simulink model "Simulink_System3"  (R2020a)
settings: Solver=VariableStepAuto  StartTime=0.0  StopTime=3  MaxStep=0.001  RelTol=1e-3
undefined symbols (not defined in the file): a, k3, kcA3, kcDO3, kcSO3, kdA3, kdDO3, kdSO3, kiA3, kiDO3, kiSO3
libraries: cstblocks x5, simulink x1
settings Model: Creator=beto1  LastModifiedBy=beto1

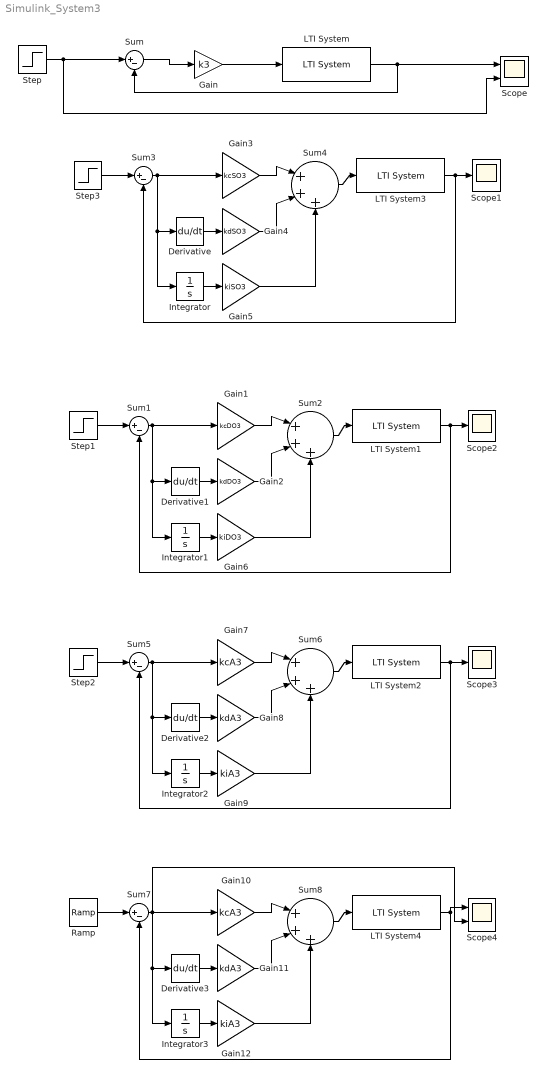
== system Simulink_System3 ==
  Derivative{,1..3} (4 alike) : Derivative
  Gain : Gain  Gain=k3
  Gain1 : Gain  Gain=kcDO3
  Gain10 : Gain  Gain=kcA3
  Gain11 : Gain  Gain=kdA3
  Gain12 : Gain  Gain=kiA3
  Gain2 : Gain  Gain=kdDO3
  Gain3 : Gain  Gain=kcSO3
  Gain4 : Gain  Gain=kdSO3
  Gain5 : Gain  Gain=kiSO3
  Gain6 : Gain  Gain=kiDO3
  Gain7 : Gain  Gain=kcA3
  Gain8 : Gain  Gain=kdA3
  Gain9 : Gain  Gain=kiA3
  Integrator{,1..3} (4 alike) : Integrator
  LTI System{,1..4} (5 alike) : cstblocks/LTI System  sys=G3  IC=[]
  Ramp : simulink/Sources/Ramp  slope=a  start=0  InitialOutput=0
  Scope : Scope  NumInputPorts=2
  Scope1 : Scope
  Scope2 : Scope
  Scope3 : Scope
  Scope4 : Scope  NumInputPorts=2
  Step : Step  Time=0  SampleTime=0
  Step1 : Step  Time=0  After=8  SampleTime=0
  Step2 : Step  Time=0  After=8  SampleTime=0
  Step3 : Step  Time=0  After=8  SampleTime=0
  Sum{,1,3,5,7} (5 alike) : Sum  Inputs=|+-
  Sum{2,4,6,8} (4 alike) : Sum  Inputs=|+++
  wires:
  Step/1 -> Sum/1, Scope/2
  LTI System/1 -> Sum/2, Scope/1
  Sum/1 -> Gain/1
  Gain/1 -> LTI System/1
  Gain4/1 -> Sum4/2
  Step3/1 -> Sum3/1
  Sum4/1 -> LTI System3/1
  Integrator/1 -> Gain5/1
  Gain5/1 -> Sum4/3
  Sum3/1 -> Integrator/1, Derivative/1, Gain3/1
  Derivative/1 -> Gain4/1
  LTI System3/1 -> Sum3/2, Scope1/1
  Gain3/1 -> Sum4/1
  Gain1/1 -> Sum2/1
  Derivative1/1 -> Gain2/1
  Integrator1/1 -> Gain6/1
  Sum2/1 -> LTI System1/1
  LTI System1/1 -> Sum1/2, Scope2/1
  Gain6/1 -> Sum2/3
  Sum1/1 -> Integrator1/1, Derivative1/1, Gain1/1
  Gain2/1 -> Sum2/2
  Step1/1 -> Sum1/1
  Sum5/1 -> Integrator2/1, Derivative2/1, Gain7/1
  Gain8/1 -> Sum6/2
  LTI System2/1 -> Sum5/2, Scope3/1
  Integrator2/1 -> Gain9/1
  Sum6/1 -> LTI System2/1
  Step2/1 -> Sum5/1
  Derivative2/1 -> Gain8/1
  Gain9/1 -> Sum6/3
  Gain7/1 -> Sum6/1
  Gain10/1 -> Sum8/1
  Integrator3/1 -> Gain12/1
  Sum8/1 -> LTI System4/1
  Gain12/1 -> Sum8/3
  Derivative3/1 -> Gain11/1
  Sum7/1 -> Scope4/2, Integrator3/1, Derivative3/1, Gain10/1
  Ramp/1 -> Sum7/1
  LTI System4/1 -> Sum7/2, Scope4/1
  Gain11/1 -> Sum8/2
